simulink model "Sistemul_neliniar"  (R2018a)
settings: Solver=VariableStepAuto  StartTime=0.0  StopTime=1.5  RelTol=1e-3
undefined symbols (not defined in the file): c1, c2, d1, d2, F1, F3, g, Jm, Jphi, Jw, k1, k3, L, m, M, R, W
settings Model: Creator=Andrei  LastModifiedBy=Andrei

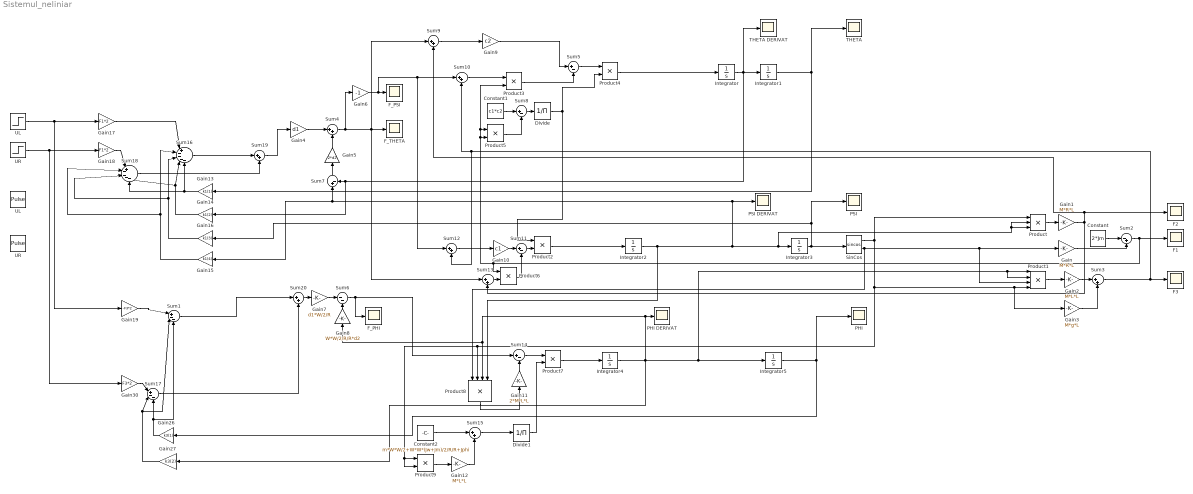
== system Sistemul_neliniar ==
  Constant : Constant  Value=2*Jm
  Constant1 : Constant  Value=c1*c2
  Constant2 : Constant  Value=m*W*W/2+W*W*(Jw+Jm)/2/R/R+Jphi
  Divide : Product  Inputs=/
  Divide1 : Product  Inputs=/
  F1 : Scope
  "F2 " : Scope
  F3 : Scope
  F_PHI : Scope
  F_PSI : Scope
  "F_THETA " : Scope
  Gain : Gain  Gain=M*R*L
  Gain1 : Gain  Gain=M*R*L
  Gain10 : Gain  Gain=c1
  Gain11 : Gain  Gain=2*M*L*L
  Gain12 : Gain  Gain=M*L*L
  Gain13 : Gain  Gain=k1(1)
  Gain14 : Gain  Gain=k1(2)
  Gain15 : Gain  Gain=k1(4)
  Gain16 : Gain  Gain=k1(3)
  Gain17 : Gain  Gain=F1*2
  Gain18 : Gain  Gain=F1*2
  Gain19 : Gain  Gain=-F3*2
  Gain2 : Gain  Gain=M*L*L
  Gain26 : Gain  Gain=k3(1)
  Gain27 : Gain  Gain=k3(2)
  Gain3 : Gain  Gain=M*g*L
  Gain30 : Gain  Gain=F3*2
  Gain4 : Gain  Gain=d1
  Gain5 : Gain  Gain=2*d2
  Gain6 : Gain  Gain=-1
  Gain7 : Gain  Gain=d1*W/2/R
  Gain8 : Gain  Gain=W*W/2/R/R*d2
  Gain9 : Gain  Gain=c2
  Integrator{,1..5} (6 alike) : Integrator
  PHI : Scope
  "PHI DERIVAT " : Scope
  "PSI " : Scope
  "PSI DERIVAT " : Scope
  Product : Product  Inputs=3
  Product1 : Product  Inputs=4
  Product{2..7,9} (7 alike) : Product
  Product8 : Product  Inputs=4
  SinCos : Trigonometry  Operator=sincos
  Sum1 : Sum  Inputs=|+--
  Sum{3..4,9..10,12..13,15,19..20} (9 alike) : Sum  Inputs=|++
  Sum{5,7..8,11,14} (5 alike) : Sum  Inputs=|+-
  Sum16 : Sum  Inputs=|+----
  Sum17 : Sum  Inputs=|+--
  Sum18 : Sum  Inputs=|+----
  Sum2 : Sum  Inputs=|-+
  Sum6 : Sum  Inputs=|--
  "THETA " : Scope
  "THETA DERIVAT " : Scope
  UL : Step  Time=0  SampleTime=0
  "UL " : DiscretePulseGenerator  PulseType=Time based  Amplitude=0.1  Period=0.02  PulseWidth=50
  UR : Step  Time=0  After=3  SampleTime=0
  "UR " : DiscretePulseGenerator  PulseType=Time based  Amplitude=1.9  Period=0.02  PulseWidth=50
  wires:
  Integrator/1 -> "THETA DERIVAT "/1, Gain14/1, Sum7/2, Integrator1/1
  Integrator1/1 -> Gain13/1, "THETA "/1
  Integrator3/1 -> SinCos/1, "PSI "/1, Gain16/1
  Integrator5/1 -> Gain26/1, PHI/1
  Integrator4/1 -> Gain27/1, Product8/3, Gain8/1, "PHI DERIVAT "/1, Product1/2, Product1/1, Integrator5/1
  UL/1 -> Gain19/1, Gain17/1
  SinCos/2 -> Product8/1, Product1/3, Gain/1
  Gain/1 -> Sum2/2
  Constant/1 -> Sum2/1
  Integrator2/1 -> Product8/4, Product/3, Product/2, Integrator3/1, "PSI DERIVAT "/1, Gain15/1, Sum7/1
  Gain1/1 -> Sum13/2, Sum9/2, "F2 "/1
  Product/1 -> Gain1/1
  Sum2/1 -> Product6/1, Product5/1, Product3/2, Product5/2, F1/1
  Product1/1 -> Gain2/1
  Gain2/1 -> Sum3/1
  Gain3/1 -> Sum3/2
  Sum3/1 -> Sum12/2, Sum10/2, F3/1
  Gain4/1 -> Sum4/1
  Gain5/1 -> Sum4/2
  Sum7/1 -> Gain5/1
  Sum4/1 -> Gain6/1, Sum9/1, Sum13/1, "F_THETA "/1
  Gain6/1 -> Sum12/1, Sum10/1, F_PSI/1
  Gain7/1 -> Sum6/1
  Gain8/1 -> Sum6/2
  Sum6/1 -> F_PHI/1, Sum14/1
  Sum9/1 -> Gain9/1
  Product3/1 -> Sum5/2
  Sum5/1 -> Product4/1
  Sum8/1 -> Divide/1
  Product5/1 -> Sum8/2
  Constant1/1 -> Sum8/1
  Divide/1 -> Product2/1, Product4/2
  Product4/1 -> Integrator/1
  Gain9/1 -> Sum5/1
  Sum10/1 -> Product3/1
  Product2/1 -> Integrator2/1
  Sum11/1 -> Product2/2
  Sum12/1 -> Gain10/1
  Gain10/1 -> Sum11/1
  Product6/1 -> Sum11/2
  Sum13/1 -> Product6/2
  Product7/1 -> Integrator4/1
  Divide1/1 -> Product7/2
  Sum14/1 -> Product7/1
  Product8/1 -> Gain11/1
  Gain11/1 -> Sum14/2
  Sum15/1 -> Divide1/1
  Constant2/1 -> Sum15/1
  Product9/1 -> Gain12/1
  Gain12/1 -> Sum15/2
  SinCos/1 -> Product/1, Gain3/1, Product1/4, Product9/1, Product9/2, Product8/2
  Gain13/1 -> Sum18/5, Sum16/5
  Gain14/1 -> Sum18/4, Sum16/4
  Gain16/1 -> Sum16/3, Sum18/3
  Gain15/1 -> Sum18/2, Sum16/2
  Gain17/1 -> Sum16/1
  Gain30/1 -> Sum17/1
  Gain26/1 -> Sum17/3, Sum1/3
  Gain27/1 -> Sum17/2, Sum1/2
  Gain18/1 -> Sum18/1
  Sum18/1 -> Sum19/2
  Sum16/1 -> Sum19/1
  Sum19/1 -> Gain4/1
  UR/1 -> Gain30/1, Gain18/1
  Gain19/1 -> Sum1/1
  Sum17/1 -> Sum20/2
  Sum20/1 -> Gain7/1
  Sum1/1 -> Sum20/1
